simulink model "thrust_weight_mass_integration"  (R2014a)
settings: Solver=ode3  StartTime=0.0  StopTime=10.0  FixedStep=0.01  RelTol=1e-3
libraries: rocket_dynamic_data_library x2
settings Model: Creator=scorpii  LastModifiedBy=scorpii

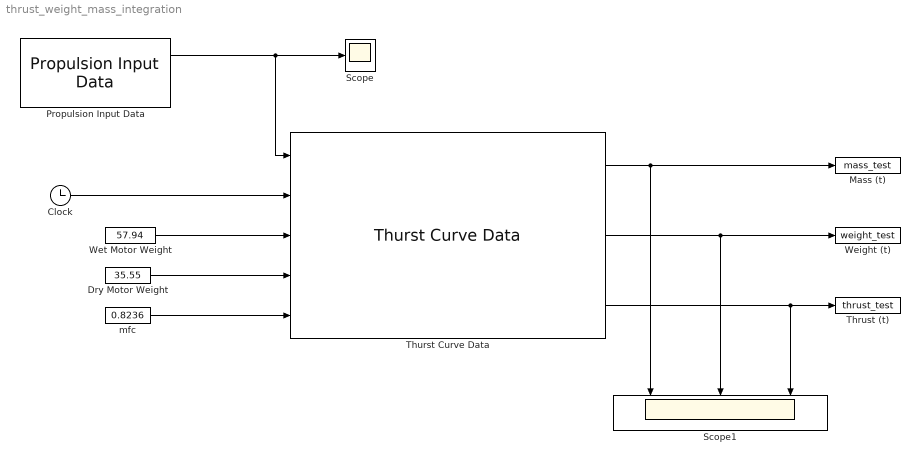
== system thrust_weight_mass_integration ==
  Clock : Clock
  Dry Motor Weight : Constant  Value=35.55
  Mass (t) : ToWorkspace  VariableName=mass_test  SampleTime=-1
  Propulsion Input Data : rocket_dynamic_data_library/Propulsion Input Data
  Scope : Scope
  Scope1 : Scope  NumInputPorts=3
      settings: YMin=-5~-5~-5  YMax=5~5~5
  Thrust (t) : ToWorkspace  VariableName=thrust_test  SampleTime=-1
  Thurst Curve Data : rocket_dynamic_data_library/Thurst Curve Data
  Weight (t) : ToWorkspace  VariableName=weight_test  SampleTime=-1
  Wet Motor Weight : Constant  Value=57.94
  mfc : Constant  Value=0.8236
  wires:
  Propulsion Input Data/1 -> Thurst Curve Data/1, Scope/1
  Clock/1 -> Thurst Curve Data/2
  Dry Motor Weight/1 -> Thurst Curve Data/4
  Wet Motor Weight/1 -> Thurst Curve Data/3
  mfc/1 -> Thurst Curve Data/5
  Thurst Curve Data/3 -> Scope1/3, Thrust (t)/1
  Thurst Curve Data/2 -> Scope1/2, Weight (t)/1
  Thurst Curve Data/1 -> Scope1/1, Mass (t)/1
